simulink model "bldc_control_speed_model"  (R2014b)
settings: Solver=ode3  StartTime=0.0  StopTime=1  FixedStep=dt  RelTol=1e-3
values from neighbouring files (symbols this model uses):
  spd_kd = 0.0    (= 0)    [bldc_control_speed_run.m]
  spd_ki = 0.002    [bldc_control_speed_run.m]
  spd_kp = 0.03    [bldc_control_speed_run.m]
  wtgt = 500*2*pi/60    (= 52.3598775598)    [bldc_control_speed_run.m]
settings Model: Creator=root  LastModifiedBy=root
settings SolverCC: AlgebraicLoopSolver=LineSearch
settings DataIOCC: LimitDataPoints=off
settings DebuggingCC: FrameProcessingCompatibilityMsg=error

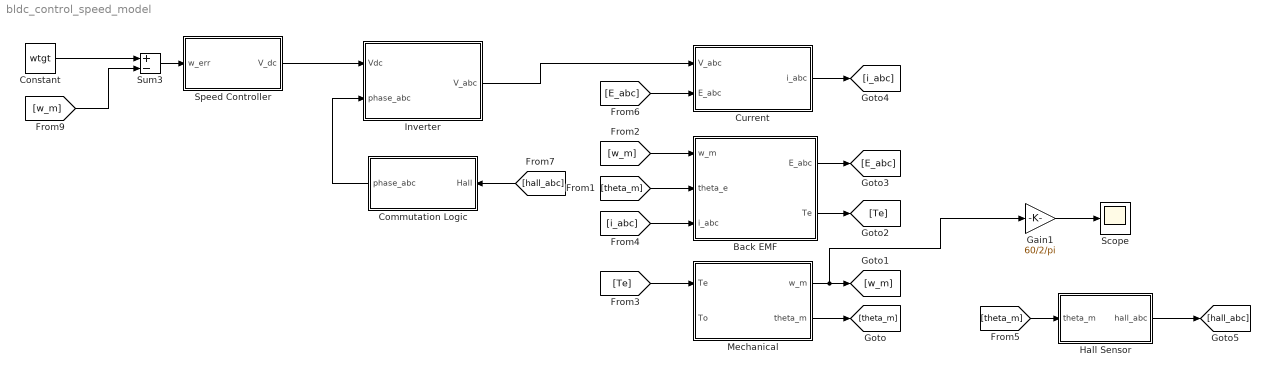
== system bldc_control_speed_model ==
  Back EMF : Subsystem
  Commutation Logic : Subsystem
  Constant : Constant  Value=wtgt
  Current : Subsystem
  Gain1 : Gain  Gain=60/2/pi
  Hall Sensor : Subsystem
  Inverter : Subsystem
  Mechanical : Subsystem
  Scope : Scope
  Speed Controller : Subsystem
  Sum3 : Sum  Inputs=+-
  wires:
  Mechanical/2(theta_m) -> [theta_m]
  Mechanical/1("w_m ") -> Gain1/1, [w_m]
  [i_abc] -> Back EMF/3(i_abc)
  [w_m] -> Back EMF/1(w_m)
  [theta_m] -> Back EMF/2(theta_e)
  Back EMF/2(Te) -> [Te]
  Back EMF/1(E_abc) -> [E_abc]
  [Te] -> Mechanical/1(Te)
  [theta_m] -> Hall Sensor/1(theta_m)
  Current/1(i_abc) -> [i_abc]
  [E_abc] -> Current/2(E_abc)
  Speed Controller/1(V_dc) -> Inverter/1(Vdc)
  Sum3/1 -> Speed Controller/1(w_err)
  Constant/1 -> Sum3/1
  [w_m] -> Sum3/2
  Inverter/1(V_abc) -> Current/1(V_abc)
  Commutation Logic/1(phase_abc) -> Inverter/2(phase_abc)
  Hall Sensor/1(hall_abc) -> [hall_abc]
  [hall_abc] -> Commutation Logic/1("Hall ")
  Gain1/1 -> Scope/1

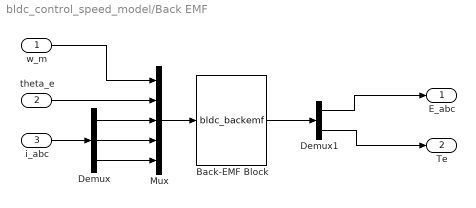
== system bldc_control_speed_model/Back EMF ==
  w_m : Inport
  theta_e : Inport  Port=2
  i_abc : Inport  Port=3
  Back-EMF Block : MATLABFcn  MATLABFcn=bldc_backemf  OutputDimensions=[4,1]  Output1D=off
  Demux : Demux  Outputs=3
  Demux1 : Demux  Outputs=[3;1]
  Mux : Mux  Inputs=5
  E_abc : Outport
  Te : Outport  Port=2
  wires:
  i_abc/1 -> Demux/1
  Demux/2 -> Mux/4
  Mux/1 -> Back-EMF Block/1
  theta_e/1 -> Mux/2
  Back-EMF Block/1 -> Demux1/1
  Demux1/1 -> E_abc/1
  Demux1/2 -> Te/1
  w_m/1 -> Mux/1
  Demux/1 -> Mux/3
  Demux/3 -> Mux/5

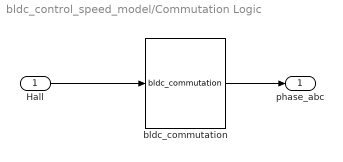
== system bldc_control_speed_model/Commutation Logic ==
  "Hall " : Inport
  bldc_commutation : MATLABFcn  MATLABFcn=bldc_commutation  OutputDimensions=[3,1]  Output1D=off
  phase_abc : Outport
  wires:
  "Hall "/1 -> bldc_commutation/1
  bldc_commutation/1 -> phase_abc/1

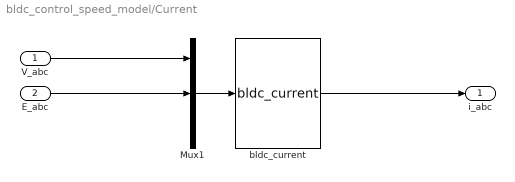
== system bldc_control_speed_model/Current ==
  V_abc : Inport
  E_abc : Inport  Port=2
  Mux1 : Mux  Inputs=[3;3;3]
  bldc_current : MATLABFcn  MATLABFcn=bldc_current  OutputDimensions=[3,1]  Output1D=off
  i_abc : Outport
  wires:
  Mux1/1 -> bldc_current/1
  E_abc/1 -> Mux1/2
  V_abc/1 -> Mux1/1
  bldc_current/1 -> i_abc/1

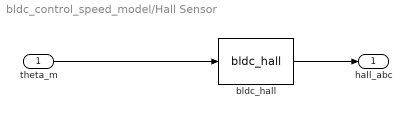
== system bldc_control_speed_model/Hall Sensor ==
  theta_m : Inport
  bldc_hall : MATLABFcn  MATLABFcn=bldc_hall  Output1D=off
  hall_abc : Outport
  wires:
  theta_m/1 -> bldc_hall/1
  bldc_hall/1 -> hall_abc/1

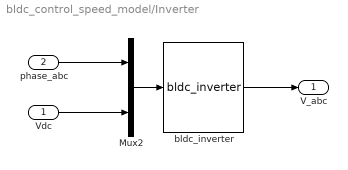
== system bldc_control_speed_model/Inverter ==
  Vdc : Inport
  phase_abc : Inport  Port=2
  Mux2 : Mux  Inputs=[3;1]
  bldc_inverter : MATLABFcn  MATLABFcn=bldc_inverter  OutputDimensions=[3,1]  Output1D=off
  V_abc : Outport
  wires:
  phase_abc/1 -> Mux2/1
  Vdc/1 -> Mux2/2
  Mux2/1 -> bldc_inverter/1
  bldc_inverter/1 -> V_abc/1

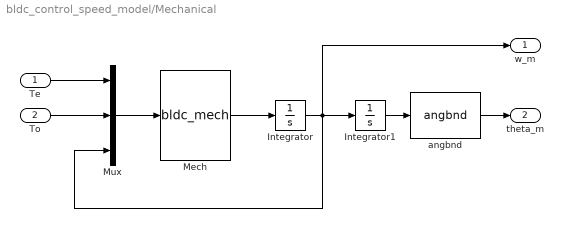
== system bldc_control_speed_model/Mechanical ==
  Te : Inport
  To : Inport  Port=2
  Integrator : Integrator
  Integrator1 : Integrator
  Mech : MATLABFcn  MATLABFcn=bldc_mech  OutputDimensions=[1,1]  Output1D=off
  Mux : Mux  Inputs=3
  angbnd : MATLABFcn  MATLABFcn=angbnd
  "w_m " : Outport
  theta_m : Outport  Port=2
  wires:
  Integrator1/1 -> angbnd/1
  Integrator/1 -> "w_m "/1, Mux/3, Integrator1/1
  Te/1 -> Mux/1
  To/1 -> Mux/2
  Mech/1 -> Integrator/1
  Mux/1 -> Mech/1
  angbnd/1 -> theta_m/1

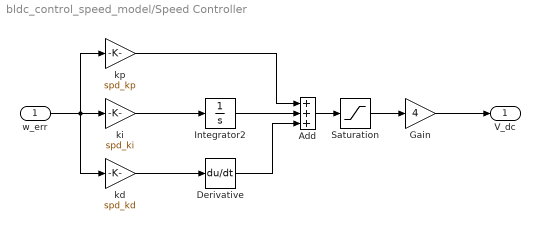
== system bldc_control_speed_model/Speed Controller ==
  w_err : Inport
  Add : Sum  Inputs=+++
  Derivative : Derivative
  Gain : Gain  Gain=4
  Integrator2 : Integrator
  Saturation : Saturate  UpperLimit=1  LowerLimit=-1
  kd : Gain  Gain=spd_kd
  ki : Gain  Gain=spd_ki
  kp : Gain  Gain=spd_kp
  V_dc : Outport
  wires:
  Add/1 -> Saturation/1
  Integrator2/1 -> Add/2
  kd/1 -> Derivative/1
  Derivative/1 -> Add/3
  ki/1 -> Integrator2/1
  kp/1 -> Add/1
  w_err/1 -> ki/1, kd/1, kp/1
  Saturation/1 -> Gain/1
  Gain/1 -> V_dc/1
